simulink model "Reg_NOnLin_14"  (Simulink 8.3)
settings: Solver=ode5  StartTime=0.0  StopTime=5  FixedStep=0.001  MaxStep=0.01  RelTol=1e-3  AbsTol=1e-3
settings Model: Creator=djemai  LastModifiedBy=szhang6_  CovHtmlReporting=off  CovSFcnEnable=on  ExtModeTrigMode=oneshot  ExtModeArmWhenConnect=off
settings DataIOCC: LimitDataPoints=off  SaveOutput=off  SaveTime=off  SignalLoggingName=sigsOut
settings OptimizationCC: BooleanDataType=off  ExpressionDepthLimit=2147483647  InitFltsAndDblsToZero=on
settings DebuggingCC: SaveWithParameterizedLinksMsg=none  SignalResolutionControl=TryResolveAllWithWarning  SolverPrmCheckMsg=none  MultiTaskDSMMsg=warning  MultiTaskCondExecSysMsg=none  FcnCallInpInsideContextMsg=EnableAllAsWarning  FrameProcessingCompatibilityMsg=error
settings HardwareCC: TargetUnknown=on
settings GRTTargetCC: TargetFcnLib=ansi_tfl_tmw.mat  GeneratePreprocessorConditionals=Use local settings

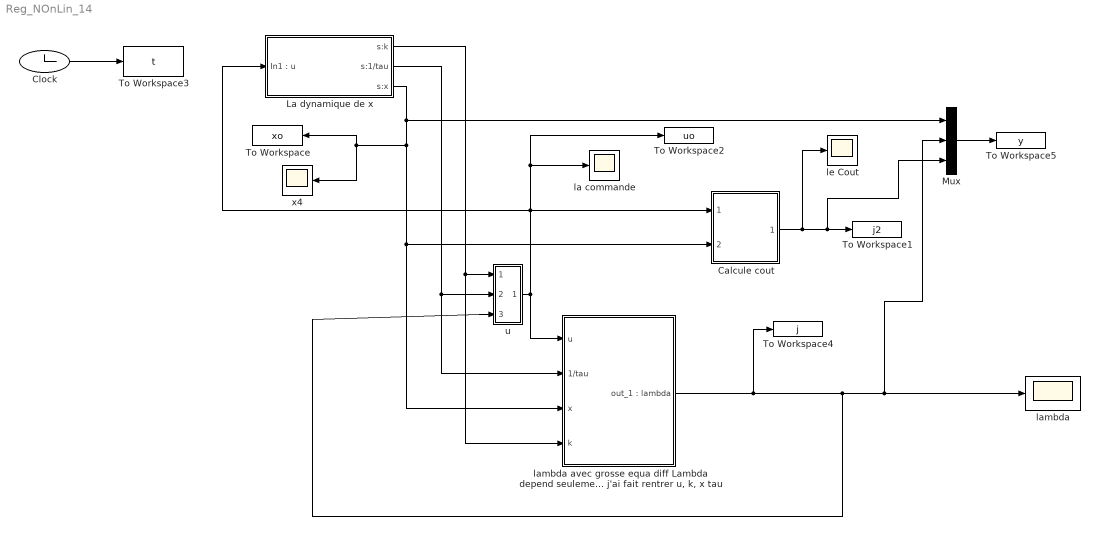
== system Reg_NOnLin_14 ==
  Calcule cout : Subsystem
  Clock : Clock
      settings: Decimation=5
  La dynamique de x : Subsystem
  Mux : Mux  Inputs=3
  To Workspace : ToWorkspace  VariableName=xo
  To Workspace1 : ToWorkspace  VariableName=j2
  To Workspace2 : ToWorkspace  VariableName=uo
  To Workspace3 : ToWorkspace  VariableName=t  SampleTime=-1
  To Workspace4 : ToWorkspace  VariableName=j
  To Workspace5 : ToWorkspace  VariableName=y
  la commande : Scope
      settings: TimeRange=5.000000  LimitDataPoints=on  MaxDataPoints=5000  SaveToWorkspace=off  SaveName=ScopeData  YMin=-1.55424  YMax=2.64978  SampleTime=-1  DataFormat=Array
  lambda : Scope
      settings: TimeRange=5.000000  LimitDataPoints=on  MaxDataPoints=5000  SaveToWorkspace=off  SaveName=ScopeData2  YMin=-2.57202  YMax=2.71074  SampleTime=-1  DataFormat=Array
  "lambda avec grosse equa diff Lambda depend seulement de x, mais pour simplifier  les sous blocs, j'ai fait rentrer u, k, x tau" : Subsystem
  le Cout : Scope
      settings: TimeRange=5.000000  LimitDataPoints=on  MaxDataPoints=5000  SaveToWorkspace=off  YMin=-1.60646  YMax=14.48098  SampleTime=-1  DataFormat=Array
  u : Subsystem
  x4 : Scope
      settings: TimeRange=5.000000  LimitDataPoints=on  MaxDataPoints=5000  SaveToWorkspace=off  SaveName=ScopeData  YMin=-0.05903  YMax=0.29479  SampleTime=-1  DataFormat=Array
  wires:
  u/1("out_1 : u") -> "lambda avec grosse equa diff Lambda depend seulement de x, mais pour simplifier  les sous blocs, j'ai fait rentrer u, k, x tau"/1(u), To Workspace2/1, la commande/1, La dynamique de x/1("In1 : u"), Calcule cout/1("in_2 : u")
  Calcule cout/1(Outport) -> Mux/3, To Workspace1/1, le Cout/1
  La dynamique de x/1(s:k) -> u/1("in_1 : k"), "lambda avec grosse equa diff Lambda depend seulement de x, mais pour simplifier  les sous blocs, j'ai fait rentrer u, k, x tau"/4(k)
  La dynamique de x/2(s:1/tau) -> "lambda avec grosse equa diff Lambda depend seulement de x, mais pour simplifier  les sous blocs, j'ai fait rentrer u, k, x tau"/2(1/tau), u/2("in_2 : 1/tau")
  La dynamique de x/3(s:x) -> To Workspace/1, x4/1, "lambda avec grosse equa diff Lambda depend seulement de x, mais pour simplifier  les sous blocs, j'ai fait rentrer u, k, x tau"/3(x), Calcule cout/2(in_1= x), Mux/1
  "lambda avec grosse equa diff Lambda depend seulement de x, mais pour simplifier  les sous blocs, j'ai fait rentrer u, k, x tau"/1("out_1 : lambda") -> u/3("in_3 : lambda"), Mux/2, lambda/1, To Workspace4/1
  Clock/1 -> To Workspace3/1
  Mux/1 -> To Workspace5/1

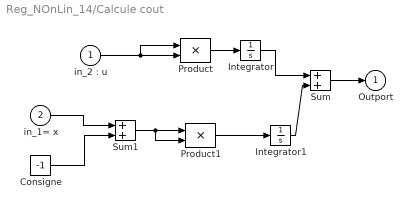
== system Reg_NOnLin_14/Calcule cout ==
  "in_2 : u" : Inport
  in_1= x : Inport  Port=2
  Consigne : Constant  Value=-1
  Integrator : Integrator
  Integrator1 : Integrator
  Product : Product  SaturateOnIntegerOverflow=on  InputSameDT=on  OutDataTypeStr=Inherit: Same as first input
  Product1 : Product  SaturateOnIntegerOverflow=on  InputSameDT=on  OutDataTypeStr=Inherit: Same as first input
  Sum : Sum  SaturateOnIntegerOverflow=on  InputSameDT=on  OutDataTypeStr=Inherit: Same as first input
  Sum1 : Sum  SaturateOnIntegerOverflow=on  InputSameDT=on  OutDataTypeStr=Inherit: Same as first input
  Outport : Outport
  wires:
  Product/1 -> Integrator/1
  Product1/1 -> Integrator1/1
  Sum/1 -> Outport/1
  Integrator/1 -> Sum/1
  Integrator1/1 -> Sum/2
  Sum1/1 -> Product1/1, Product1/2
  in_1= x/1 -> Sum1/1
  "in_2 : u"/1 -> Product/2, Product/1
  Consigne/1 -> Sum1/2

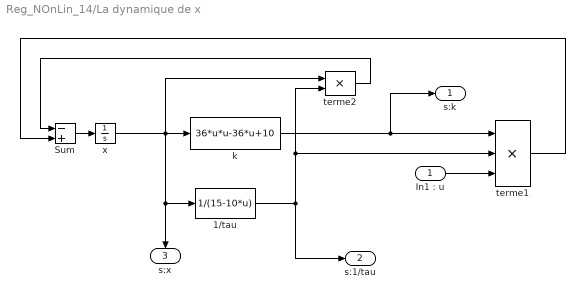
== system Reg_NOnLin_14/La dynamique de x ==
  "In1 : u" : Inport
  1/tau : Fcn  Expr=1/(15-10*u)
  Sum : Sum  Inputs=-+  SaturateOnIntegerOverflow=on  InputSameDT=on  OutDataTypeStr=Inherit: Same as first input
  k : Fcn  Expr=36*u*u-36*u+10
  terme1 : Product  Inputs=3  SaturateOnIntegerOverflow=on  InputSameDT=on  OutDataTypeStr=Inherit: Same as first input
  terme2 : Product  SaturateOnIntegerOverflow=on  InputSameDT=on  OutDataTypeStr=Inherit: Same as first input
  x : Integrator
  s:k : Outport
  s:1/tau : Outport  Port=2
  s:x : Outport  Port=3
  wires:
  x/1 -> terme2/1, s:x/1, 1/tau/1, k/1
  1/tau/1 -> terme2/2, terme1/2, s:1/tau/1
  terme2/1 -> Sum/1
  terme1/1 -> Sum/2
  Sum/1 -> x/1
  "In1 : u"/1 -> terme1/3
  k/1 -> s:k/1, terme1/1

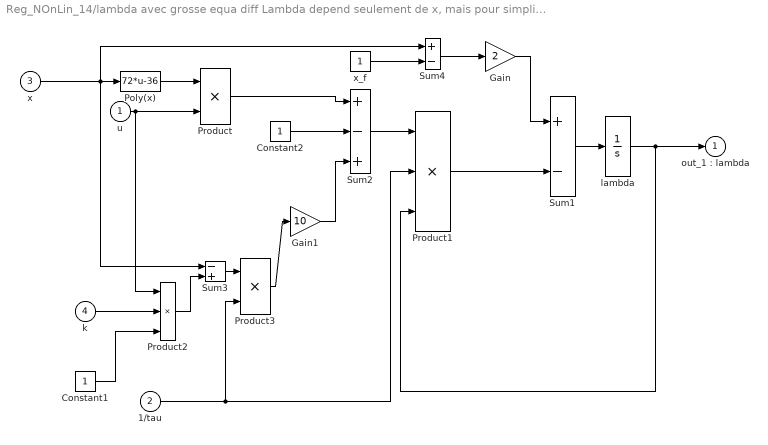
== system Reg_NOnLin_14/lambda avec grosse equa diff Lambda depend seulement de x, mais pour simplifier  les sous blocs, j'ai fait rentrer u, k, x tau ==
  u : Inport
  1/tau : Inport  Port=2
  x : Inport  Port=3
  k : Inport  Port=4
  Constant1 : Constant
  Constant2 : Constant
  Gain : Gain  Gain=2  SaturateOnIntegerOverflow=on  OutDataTypeStr=Inherit: Same as input  ParamDataTypeStr=Inherit: Same as input
  Gain1 : Gain  Gain=10  SaturateOnIntegerOverflow=on  OutDataTypeStr=Inherit: Same as input  ParamDataTypeStr=Inherit: Same as input
  Poly(x) : Fcn  Expr=72*u-36
  Product : Product  SaturateOnIntegerOverflow=on  InputSameDT=on  OutDataTypeStr=Inherit: Same as first input
  Product1 : Product  Inputs=3  SaturateOnIntegerOverflow=on  InputSameDT=on  OutDataTypeStr=Inherit: Same as first input
  Product2 : Product  Inputs=3  SaturateOnIntegerOverflow=on  InputSameDT=on  OutDataTypeStr=Inherit: Same as first input
  Product3 : Product  SaturateOnIntegerOverflow=on  InputSameDT=on  OutDataTypeStr=Inherit: Same as first input
  Sum1 : Sum  Inputs=+-  SaturateOnIntegerOverflow=on  InputSameDT=on  OutDataTypeStr=Inherit: Same as first input
  Sum2 : Sum  Inputs=+-+  SaturateOnIntegerOverflow=on  InputSameDT=on  OutDataTypeStr=Inherit: Same as first input
  Sum3 : Sum  Inputs=-+  SaturateOnIntegerOverflow=on  InputSameDT=on  OutDataTypeStr=Inherit: Same as first input
  Sum4 : Sum  Inputs=+-  SaturateOnIntegerOverflow=on  InputSameDT=on  OutDataTypeStr=Inherit: Same as first input
  lambda : Integrator  InitialCondition=2
  x_f : Constant
  "out_1 : lambda" : Outport
  wires:
  Sum2/1 -> Product1/1
  Product/1 -> Sum2/1
  x/1 -> Poly(x)/1, Sum4/1, Sum3/1
  Sum1/1 -> lambda/1
  Gain/1 -> Sum1/1
  lambda/1 -> "out_1 : lambda"/1, Product1/3
  Product1/1 -> Sum1/2
  Poly(x)/1 -> Product/1
  u/1 -> Product/2, Product2/1
  1/tau/1 -> Product1/2, Product3/2
  k/1 -> Product2/2
  Constant1/1 -> Product2/3
  Product2/1 -> Sum3/2
  Sum3/1 -> Product3/1
  Product3/1 -> Gain1/1
  Constant2/1 -> Sum2/2
  Gain1/1 -> Sum2/3
  x_f/1 -> Sum4/2
  Sum4/1 -> Gain/1

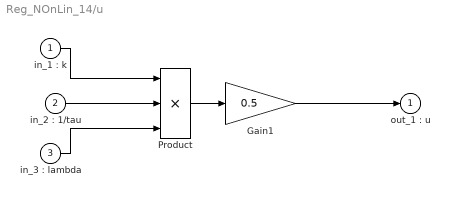
== system Reg_NOnLin_14/u ==
  "in_1 : k" : Inport
  "in_2 : 1/tau" : Inport  Port=2
  "in_3 : lambda" : Inport  Port=3
  Gain1 : Gain  Gain=0.5  SaturateOnIntegerOverflow=on  OutDataTypeStr=Inherit: Same as input  ParamDataTypeStr=Inherit: Same as input
  Product : Product  Inputs=3  SaturateOnIntegerOverflow=on  InputSameDT=on  OutDataTypeStr=Inherit: Same as first input
  "out_1 : u" : Outport
  wires:
  Product/1 -> Gain1/1
  "in_1 : k"/1 -> Product/1
  "in_2 : 1/tau"/1 -> Product/2
  Gain1/1 -> "out_1 : u"/1
  "in_3 : lambda"/1 -> Product/3
